simulink model "jib_model"  (Simulink 7.8)
settings: Solver=VariableStepDiscrete  StartTime=0.0  StopTime=10.0  RelTol=1e-3
undefined symbols (not defined in the file): jib, jib_x0, jib_xref, Ts
libraries: simulink x1
settings Model: Creator=matias  LastModifiedBy=UCH
settings GRTTargetCC: CombineOutputUpdateFcns=on

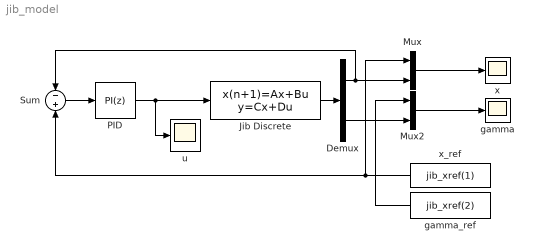
== system jib_model ==
  Demux : Demux  Outputs=2
  Jib Discrete : DiscreteStateSpace  A=jib.A  B=jib.B  C=jib.C  D=jib.D  X0=jib_x0  SampleTime=Ts
  Mux : Mux  Inputs=2
  Mux2 : Mux  Inputs=2
  PID : simulink/Continuous/PID Controller  Controller=PI  TimeDomain=Discrete-time  SampleTime=Ts  IntegratorMethod=Forward Euler  FilterMethod=Forward Euler  Form=Parallel  P=1  I=1  D=0  N=0  InitialConditionSource=internal  InitialConditionForIntegrator=0  InitialConditionForFilter=0  ExternalReset=none  LimitOutput=off  UpperSaturationLimit=1  LowerSaturationLimit=-1  LinearizeAsGain=off  AntiWindupMode=clamping  Kb=1  TrackingMode=off  Kt=1  PParamMin=[]  PParamMax=[]  IParamMin=[]  IParamMax=[]  DParamMin=[]  DParamMax=[]  NParamMin=[]  NParamMax=[]  KbParamMin=[]  KbParamMax=[]  KtParamMin=[]  KtParamMax=[]  POutMin=[]  POutMax=[]  IOutMin=[]  IOutMax=[]  DOutMin=[]  DOutMax=[]  NOutMin=[]  NOutMax=[]  KbOutMin=[]  KbOutMax=[]  KtOutMin=[]  KtOutMax=[]  IntegratorOutMin=[]  IntegratorOutMax=[]  FilterOutMin=[]  FilterOutMax=[]  SumOutMin=[]  SumOutMax=[]  SumI1OutMin=[]  SumI1OutMax=[]  SumI2OutMin=[]  SumI2OutMax=[]  SumI3OutMin=[]  SumI3OutMax=[]  SumDOutMin=[]  SumDOutMax=[]  SaturationOutMin=[]  SaturationOutMax=[]  IntegratorContinuousStateAttributes=''  IntegratorStateMustResolveToSignalObject=off  IntegratorRTWStateStorageClass=Auto  FilterContinuousStateAttributes=''  FilterStateMustResolveToSignalObject=off  FilterRTWStateStorageClass=Auto
  Sum : Sum  Inputs=-|+  SampleTime=Ts
  gamma : Scope
      settings: TimeRange=10
  gamma_ref : Constant  Value=jib_xref(2)
  u : Scope
      settings: YMin=-5500  YMax=6000  SaveName=ScopeData2
  x : Scope
      settings: YMin=-220  YMax=10
  x_ref : Constant  Value=jib_xref(1)
  wires:
  Jib Discrete/1 -> Demux/1
  Mux/1 -> x/1
  Mux2/1 -> gamma/1
  Demux/1 -> Mux/2, Sum/1
  Demux/2 -> Mux2/2
  Sum/1 -> PID/1
  PID/1 -> Jib Discrete/1, u/1
  x_ref/1 -> Mux/1, Sum/2
  gamma_ref/1 -> Mux2/1
